simulink model "Composition"  (R2023a)
settings: Solver=FixedStepDiscrete  StartTime=0.0  StopTime=10.0  FixedStep=Ts  RelTol=1e-3
PostLoadFcn:
  | HBridgeCmd_LkupTbl = Simulink.LookupTable;
  | HBridgeCmd_LkupTbl.Table.DataType = 'int16';
  | HBridgeCmd_LkupTbl.Table.Min = [];
  | HBridgeCmd_LkupTbl.Table.Max = [];
  | HBridgeCmd_LkupTbl.Table.Unit = '';
  | HBridgeCmd_LkupTbl.Table.FieldName = 'Table';
  | HBridgeCmd_LkupTbl.Table.Description = '';
  | HBridgeCmd_LkupTbl.Table.Value = int16( ...
  |   [-2048 -1843 -1638 -1434 -1229 -1024 -819 -614 -410 -205 0 205 410 614 ...
  |    819 1024 1229 1434 1638 1843 2048]);
  | HBridgeCmd_LkupTbl.BreakpointsSpecification = 'Explicit values';
  | HBridgeCmd_LkupTbl.SupportTunableSize = false;
  | HBridgeCmd_LkupTbl.Breakpoints.DataType = 'single';
  | HBridgeCmd_LkupTbl.Breakpoints.Min = [];
  | HBridgeCmd_LkupTbl.Breakpoints.Max = [];
  | HBridgeCmd_LkupTbl.Breakpoints.Unit = '';
  | HBridgeCmd_LkupTbl.Breakpoints.FieldName = 'BP1';
  | HBridgeCmd_LkupTbl.Breakpoints.Description = '';
  | HBridgeCmd_LkupTbl.Breakpoints.Value = ...
  |   [-100 -90 -80 -70 -60 -50 -40 -30 -20 -10 0 10 20 30 40 50 60 70 80 90 ...
  |    100];
  | HBridgeCmd_LkupTbl.Breakpoints.TunableSizeName = 'N1';
  | HBridgeCmd_LkupTbl.CoderInfo.StorageClass = 'Auto';
  | HBridgeCmd_LkupTbl.StructTypeInfo.Name = 'MyStruct_Actuator';
  | HBridgeCmd_LkupTbl.StructTypeInfo.DataScope = 'Auto';
  | HBridgeCmd_LkupTbl.StructTypeInfo.HeaderFileName = '';
  | 
  | APP_FilterWeight = Simulink.Parameter;
  | APP_FilterWeight.Value = 1;
  | APP_FilterWeight.CoderInfo.StorageClass = 'Auto';
  | APP_FilterWeight.Description = '';
  | APP_FilterWeight.DataType = 'single';
  | APP_FilterWeight.Min = 0;
  | APP_FilterWeight.Max = 1;
  | APP_FilterWeight.DocUnits = '';
  | 
  | TPS_Primary_FilterWeight = Simulink.Parameter;
  | TPS_Primary_FilterWeight.Value = 1;
  | TPS_Primary_FilterWeight.CoderInfo.StorageClass = 'Auto';
  | TPS_Primary_FilterWeight.Description = '';
  | TPS_Primary_FilterWeight.DataType = 'single';
  | TPS_Primary_FilterWeight.Min = 0;
  | TPS_Primary_FilterWeight.Max = 1;
  | TPS_Primary_FilterWeight.DocUnits = '';
  | 
  | TPS_Secondary_FilterWeight = Simulink.Parameter;
  | TPS_Secondary_FilterWeight.Value = 1;
  | TPS_Secondary_FilterWeight.CoderInfo.StorageClass = 'Auto';
  | TPS_Secondary_FilterWeight.Description = '';
  | TPS_Secondary_FilterWeight.DataType = 'single';
  | TPS_Secondary_FilterWeight.Min = 0;
  | TPS_Secondary_FilterWeight.Max = 1;
  | TPS_Secondary_FilterWeight.DocUnits = '';
  | 
  | AccelPedal_Threshold_High = Simulink.Parameter;
  | AccelPedal_Threshold_High.Value = 975;
  | AccelPedal_Threshold_High.CoderInfo.StorageClass = 'Auto';
  | AccelPedal_Threshold_High.Description = '';
  | AccelPedal_Threshold_High.DataType = 'uint16';
  | AccelPedal_Threshold_High.Min = 0;
  | AccelPedal_Threshold_High.Max = 1023;
  | AccelPedal_Threshold_High.DocUnits = '';
  | 
  | AccelPedal_Threshold_Low = Simulink.Parameter;
  | AccelPedal_Threshold_Low.Value = 50;
  | AccelPedal_Threshold_Low.CoderInfo.StorageClass = 'Auto';
  | AccelPedal_Threshold_Low.Description = '';
  | AccelPedal_Threshold_Low.DataType = 'uint16';
  | AccelPedal_Threshold_Low.Min = 0;
  | AccelPedal_Threshold_Low.Max = 1023;
  | AccelPedal_Threshold_Low.DocUnits = '';
  | 
  | TPS_Primary_Threshold_High = Simulink.Parameter;
  | TPS_Primary_Threshold_High.Value = 975;
  | TPS_Primary_Threshold_High.CoderInfo.StorageClass = 'Auto';
  | TPS_Primary_Threshold_High.Description = '';
  | TPS_Primary_Threshold_High.DataType = 'uint16';
  | TPS_Primary_Threshold_High.Min = 0;
  | TPS_Primary_Threshold_High.Max = 1023;
  | TPS_Primary_Threshold_High.DocUnits = '';
  | 
  | TPS_Primary_Threshold_Low = Simulink.Parameter;
  | TPS_Primary_Threshold_Low.Value = 50;
  | TPS_Primary_Threshold_Low.CoderInfo.StorageClass = 'Auto';
  | TPS_Primary_Threshold_Low.Description = '';
  | TPS_Primary_Threshold_Low.DataType = 'uint16';
  | TPS_Primary_Threshold_Low.Min = 0;
  | TPS_Primary_Threshold_Low.Max = 1023;
  | TPS_Primary_Threshold_Low.DocUnits = '';
  | 
  | TPS_Secondary_Threshold_High = Simulink.Parameter;
  | TPS_Secondary_Threshold_High.Value = 975;
  | TPS_Secondary_Threshold_High.CoderInfo.StorageClass = 'Auto';
  | TPS_Secondary_Threshold_High.Description = '';
  | TPS_Secondary_Threshold_High.DataType = 'uint16';
  | TPS_Secondary_Threshold_High.Min = 0;
  | TPS_Secondary_Threshold_High.Max = 1023;
  | TPS_Secondary_Threshold_High.DocUnits = '';
  | 
  | TPS_Secondary_Threshold_Low = Simulink.Parameter;
  | TPS_Secondary_Threshold_Low.Value = 50;
  | TPS_Secondary_Threshold_Low.CoderInfo.StorageClass = 'Auto';
  | TPS_Secondary_Threshold_Low.Description = '';
  | TPS_Secondary_Threshold_Low.DataType = 'uint16';
  | TPS_Secondary_Threshold_Low.Min = 0;
  | TPS_Secondary_Threshold_Low.Max = 1023;
  | TPS_Secondary_Threshold_Low.DocUnits = '';
  | 
  | 
  | SetpointPercent_LkupTbl = Simulink.LookupTable;
  | SetpointPercent_LkupTbl.Table.DataType = 'single';
  | SetpointPercent_LkupTbl.Table.Min = [];
  | SetpointPercent_LkupTbl.Table.Max = [];
  | SetpointPercent_LkupTbl.Table.Unit = '';
  | SetpointPercent_LkupTbl.Table.FieldName = 'Table';
  | SetpointPercent_LkupTbl.Table.Description = '';
  | SetpointPercent_LkupTbl.Table.Value = ...
  |   [0 10 20 30 40 50 60 70 80 90 100];
  | SetpointPercent_LkupTbl.BreakpointsSpecification = 'Explicit values';
  | SetpointPercent_LkupTbl.SupportTunableSize = false;
  | SetpointPercent_LkupTbl.Breakpoints.DataType = 'single';
  | SetpointPercent_LkupTbl.Breakpoints.Min = [];
  | SetpointPercent_LkupTbl.Breakpoints.Max = [];
  | SetpointPercent_LkupTbl.Breakpoints.Unit = '';
  | SetpointPercent_LkupTbl.Breakpoints.FieldName = 'BP1';
  | SetpointPercent_LkupTbl.Breakpoints.Description = '';
  | SetpointPercent_LkupTbl.Breakpoints.Value = ...
  |   [0 100 200 300 400 500 600 700 800 900 1000];
  | SetpointPercent_LkupTbl.Breakpoints.TunableSizeName = 'N1';
  | SetpointPercent_LkupTbl.CoderInfo.StorageClass = 'Auto';
  | SetpointPercent_LkupTbl.StructTypeInfo.Name = 'MyStruct';
  | SetpointPercent_LkupTbl.StructTypeInfo.DataScope = 'Auto';
  | SetpointPercent_LkupTbl.StructTypeInfo.HeaderFileName = '';
  | 
  | TPSPrimaryPercent_LkupTbl = Simulink.LookupTable;
  | TPSPrimaryPercent_LkupTbl.Table.DataType = 'single';
  | TPSPrimaryPercent_LkupTbl.Table.Min = [];
  | TPSPrimaryPercent_LkupTbl.Table.Max = [];
  | TPSPrimaryPercent_LkupTbl.Table.Unit = '';
  | TPSPrimaryPercent_LkupTbl.Table.FieldName = 'Table';
  | TPSPrimaryPercent_LkupTbl.Table.Description = '';
  | TPSPrimaryPercent_LkupTbl.Table.Value = ...
  |   [0 10 20 30 40 50 60 70 80 90 100];
  | TPSPrimaryPercent_LkupTbl.BreakpointsSpecification = 'Explicit values';
  | TPSPrimaryPercent_LkupTbl.SupportTunableSize = false;
  | TPSPrimaryPercent_LkupTbl.Breakpoints.DataType = 'single';
  | TPSPrimaryPercent_LkupTbl.Breakpoints.Min = [];
  | TPSPrimaryPercent_LkupTbl.Breakpoints.Max = [];
  | TPSPrimaryPercent_LkupTbl.Breakpoints.Unit = '';
  | TPSPrimaryPercent_LkupTbl.Breakpoints.FieldName = 'BP1';
  | TPSPrimaryPercent_LkupTbl.Breakpoints.Description = '';
  | TPSPrimaryPercent_LkupTbl.Breakpoints.Value = ...
  |   [0 100 200 300 400 500 600 700 800 900 1000];
  | TPSPrimaryPercent_LkupTbl.Breakpoints.TunableSizeName = 'N1';
  | TPSPrimaryPercent_LkupTbl.CoderInfo.StorageClass = 'Auto';
  | TPSPrimaryPercent_LkupTbl.StructTypeInfo.Name = 'MyStruct';
  | TPSPrimaryPercent_LkupTbl.StructTypeInfo.DataScope = 'Auto';
  | TPSPrimaryPercent_LkupTbl.StructTypeInfo.HeaderFileName = '';
  | 
  | TPSSecondaryPercent_LkupTbl = Simulink.LookupTable;
  | TPSSecondaryPercent_LkupTbl.Table.DataType = 'single';
  | TPSSecondaryPercent_LkupTbl.Table.Min = [];
  | TPSSecondaryPercent_LkupTbl.Table.Max = [];
  | TPSSecondaryPercent_LkupTbl.Table.Unit = '';
  | TPSSecondaryPercent_LkupTbl.Table.FieldName = 'Table';
  | TPSSecondaryPercent_LkupTbl.Table.Description = '';
  | TPSSecondaryPercent_LkupTbl.Table.Value = ...
  |   [100 90 80 70 60 50 40 30 20 10 0];
  | TPSSecondaryPercent_LkupTbl.BreakpointsSpecification = ...
  |   'Explicit values';
  | TPSSecondaryPercent_LkupTbl.SupportTunableSize = false;
  | TPSSecondaryPercent_LkupTbl.Breakpoints.DataType = 'single';
  | TPSSecondaryPercent_LkupTbl.Breakpoints.Min = [];
  | TPSSecondaryPercent_LkupTbl.Breakpoints.Max = [];
  | TPSSecondaryPercent_LkupTbl.Breakpoints.Unit = '';
  | TPSSecondaryPercent_LkupTbl.Breakpoints.FieldName = 'BP1';
  | TPSSecondaryPercent_LkupTbl.Breakpoints.Description = '';
  | TPSSecondaryPercent_LkupTbl.Breakpoints.Value = ...
  |   [0 100 200 300 400 500 600 700 800 900 1000];
  | TPSSecondaryPercent_LkupTbl.Breakpoints.TunableSizeName = 'N1';
  | TPSSecondaryPercent_LkupTbl.CoderInfo.StorageClass = 'Auto';
  | TPSSecondaryPercent_LkupTbl.StructTypeInfo.Name = 'MyStruct';
  | TPSSecondaryPercent_LkupTbl.StructTypeInfo.DataScope = 'Auto';
  | TPSSecondaryPercent_LkupTbl.StructTypeInfo.HeaderFileName = '';
  | 
  | Ts = 0.005;
undefined symbols (not defined in the file): D1, P
CloseFcn:
  | clear Ts TPSSecondaryPercent_LkupTbl TPSPrimaryPercent_LkupTbl SetpointPercent_LkupTbl ...
  |     TPS_Secondary_Threshold_High TPS_Secondary_Threshold_Low ...
  |     TPS_Primary_Threshold_High TPS_Primary_Threshold_Low ...
  |     TPS_Primary_FilterWeight TPS_Secondary_FilterWeight ...
  |     AccelPedal_Threshold_High AccelPedal_Threshold_Low ...
  |     APP_FilterWeight HBridgeCmd_LkupTbl
settings Model: Creator=The MathWorks, Inc.  LastModifiedBy=omert
settings OptimizationCC: DefaultParameterBehavior=Inlined  EnhancedBackFolding=on  PassReuseOutputArgsAs=Individual arguments  ZeroExternalMemoryAtStartup=off  ZeroInternalMemoryAtStartup=off  OptimizeBlockOrder=speed  DifferentSizesBufferReuse=on  OptimizationCustomize=off  EfficientTunableParamExpr=on
settings DebuggingCC: ParameterTunabilityLossMsg=error  UnconnectedInputMsg=warning  UnconnectedOutputMsg=warning  UnconnectedLineMsg=warning
settings ModelReferenceCC: EnableRefExpFcnMdlSchedulingChecks=on
settings SFSimCC: MATLABDynamicMemAlloc=off
settings RTWCC: Description=Embedded Coder  SystemTargetFile=ert.tlc  TemplateMakefile=ert_default_tmf  DLArmComputeVersion=19.05
settings CodeAppCC: ForceParamTrailComments=on  IgnoreCustomStorageClasses=off  MaxIdLength=255  OperatorAnnotations=on  SimulinkDataObjDesc=on  SFDataObjDesc=on  InsertBlockDesc=on
settings ERTTargetCC: TargetLangStandard=C99 (ISO)  GenerateSampleERTMain=on  InlinedParameterPlacement=NonHierarchical  ERTCustomFileTemplate=example_file_process.tlc

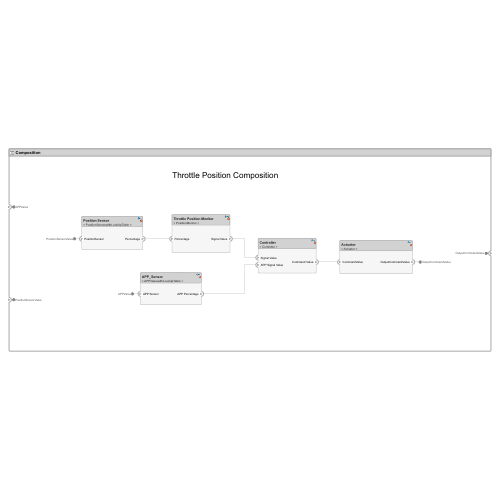
[thumbnail: Simulink's stored preview of the top-level diagram]
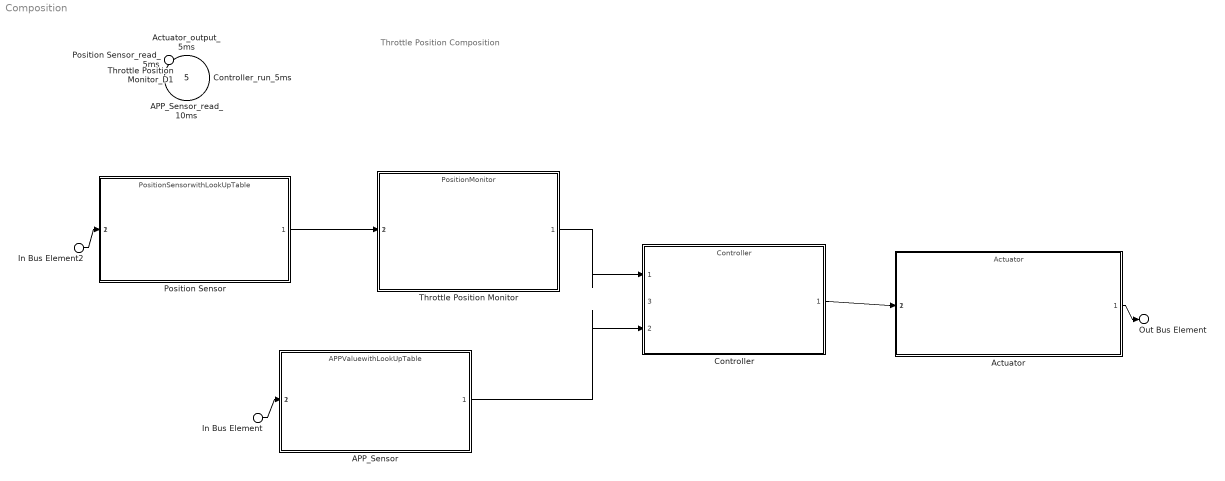
== system Composition ==
  note: Throttle Position Composition
  In Bus Element : Inport  PortName=APPValue
  In Bus Element2 : Inport  Port=2  PortName=PositionSensorValue
  APP_Sensor_read_10ms : Inport  Port=3  OutputFunctionCall=on
  Actuator_output_5ms : Inport  Port=4  OutputFunctionCall=on
  Controller_run_5ms : Inport  Port=5  OutputFunctionCall=on
  Position Sensor_read_5ms : Inport  Port=6  OutputFunctionCall=on
  Throttle Position Monitor_D1 : Inport  Port=7  OutputFunctionCall=on
  APP_Sensor : ModelReference  ModelNameDialog=APPValuewithLookUpTable  SimulationMode=Normal  ScheduleRates=on  ModelReferenceVersion=5.2
      settings: PortSchema="{\"entries\":[{\"content\":{\"headerSize\":38,\"margin\":15,\"minimumSpacing\":25,\"sides\":[{\"content\":{\"connectorIds\":[\"In1\"]},\"type\":\"ConnectorPlacement.EquallySpacedRectSide\",\"uuid\":\"c29aa152-21e6-4ee4-993c-b72c52d53eaf\"},{\"content\":{\"connectorIds\":[\"Out1\"],\"side\":\"RIGHT\"},\"type\":\"ConnectorPlacement.EquallySpacedRectSide\",\"uuid\":\"9c4e8262-d4f5-4a71-85d6-4174f9813a5f\"},{\"content\":{\"connectorIds\":[],\"side\":\"TOP\"},\"type\":\"ConnectorPlacement.EquallySpacedRectSide\",\"uuid\":\"c9ef3685-fbcc-4180-9c44-6a6e7c5f1244\"},{\"content\":{\"connectorIds\":[\"In2\"],\"side\":\"HIDDEN\"},\"type\":\"ConnectorPlacement.EquallySpacedRectSide\",\"uuid\":\"f1270cb8-53b9-476f-b22e-76ae4b133e3f\"}]},\"type\":\"ConnectorPlacement.EquallySpacedConnector\",\"uuid\":\"93ccf44c-7afb-4857-9748-e933214d86ea\"}],\"packageUris\":[\"http://schema.mathworks.com/mf0/Connector/R2020b\"],\"version\":\"1.0\"}"
  Actuator : ModelReference  ModelNameDialog=Actuator  SimulationMode=Normal  ScheduleRates=on  ModelReferenceVersion=5.2
      settings: PortSchema="{\"entries\":[{\"content\":{\"headerSize\":38,\"margin\":15,\"minimumSpacing\":25,\"sides\":[{\"content\":{\"connectorIds\":[\"In1\"]},\"type\":\"ConnectorPlacement.EquallySpacedRectSide\",\"uuid\":\"c29aa152-21e6-4ee4-993c-b72c52d53eaf\"},{\"content\":{\"connectorIds\":[\"Out1\"],\"side\":\"RIGHT\"},\"type\":\"ConnectorPlacement.EquallySpacedRectSide\",\"uuid\":\"9c4e8262-d4f5-4a71-85d6-4174f9813a5f\"},{\"content\":{\"connectorIds\":[],\"side\":\"TOP\"},\"type\":\"ConnectorPlacement.EquallySpacedRectSide\",\"uuid\":\"c9ef3685-fbcc-4180-9c44-6a6e7c5f1244\"},{\"content\":{\"connectorIds\":[\"In2\"],\"side\":\"HIDDEN\"},\"type\":\"ConnectorPlacement.EquallySpacedRectSide\",\"uuid\":\"00201e36-4798-4d6f-9c06-922f886f8b8e\"}]},\"type\":\"ConnectorPlacement.EquallySpacedConnector\",\"uuid\":\"93ccf44c-7afb-4857-9748-e933214d86ea\"}],\"packageUris\":[\"http://schema.mathworks.com/mf0/Connector/R2020b\"],\"version\":\"1.0\"}"
  Controller : ModelReference  ModelNameDialog=Controller  SimulationMode=Normal  ScheduleRates=on  ModelReferenceVersion=5.4
      settings: PortSchema="{\"entries\":[{\"content\":{\"headerSize\":38,\"margin\":15,\"minimumSpacing\":25,\"sides\":[{\"content\":{\"connectorIds\":[\"In1\",\"In2\"]},\"type\":\"ConnectorPlacement.EquallySpacedRectSide\",\"uuid\":\"c29aa152-21e6-4ee4-993c-b72c52d53eaf\"},{\"content\":{\"connectorIds\":[\"Out1\"],\"side\":\"RIGHT\"},\"type\":\"ConnectorPlacement.EquallySpacedRectSide\",\"uuid\":\"9c4e8262-d4f5-4a71-85d6-4174f9813a5f\"},{\"content\":{\"connectorIds\":[],\"side\":\"TOP\"},\"type\":\"ConnectorPlacement.EquallySpacedRectSide\",\"uuid\":\"c9ef3685-fbcc-4180-9c44-6a6e7c5f1244\"},{\"content\":{\"connectorIds\":[\"In3\"],\"side\":\"HIDDEN\"},\"type\":\"ConnectorPlacement.EquallySpacedRectSide\",\"uuid\":\"cd41997d-1e34-4368-8511-2b1fe694f98a\"}]},\"type\":\"ConnectorPlacement.EquallySpacedConnector\",\"uuid\":\"93ccf44c-7afb-4857-9748-e933214d86ea\"}],\"packageUris\":[\"http://schema.mathworks.com/mf0/Connector/R2020b\"],\"version\":\"1.0\"}"
  Position Sensor : ModelReference  ModelNameDialog=PositionSensorwithLookUpTable  UsingDefaultArgumentValue=0  SimulationMode=Normal  ScheduleRates=on  ModelReferenceVersion=5.3
      settings: PortSchema="{\"entries\":[{\"content\":{\"headerSize\":38,\"margin\":15,\"minimumSpacing\":25,\"sides\":[{\"content\":{\"connectorIds\":[\"In1\"]},\"type\":\"ConnectorPlacement.EquallySpacedRectSide\",\"uuid\":\"c29aa152-21e6-4ee4-993c-b72c52d53eaf\"},{\"content\":{\"connectorIds\":[\"Out1\"],\"side\":\"RIGHT\"},\"type\":\"ConnectorPlacement.EquallySpacedRectSide\",\"uuid\":\"9c4e8262-d4f5-4a71-85d6-4174f9813a5f\"},{\"content\":{\"connectorIds\":[],\"side\":\"TOP\"},\"type\":\"ConnectorPlacement.EquallySpacedRectSide\",\"uuid\":\"c9ef3685-fbcc-4180-9c44-6a6e7c5f1244\"},{\"content\":{\"connectorIds\":[\"In2\"],\"side\":\"HIDDEN\"},\"type\":\"ConnectorPlacement.EquallySpacedRectSide\",\"uuid\":\"9e42063d-e5ff-4629-a071-cb979e3a0f50\"}]},\"type\":\"ConnectorPlacement.EquallySpacedConnector\",\"uuid\":\"93ccf44c-7afb-4857-9748-e933214d86ea\"}],\"packageUris\":[\"http://schema.mathworks.com/mf0/Connector/R2020b\"],\"version\":\"1.0\"}"
  Throttle Position Monitor : ModelReference  ModelNameDialog=PositionMonitor  SimulationMode=Normal  ScheduleRates=on  CachedPortDiscreteRates=[0.005]  ModelEventPortInfo=P:D1[0.005][0][0]  ModelReferenceVersion=5.2
      settings: PortSchema="{\"entries\":[{\"content\":{\"headerSize\":38,\"margin\":15,\"minimumSpacing\":25,\"sides\":[{\"content\":{\"connectorIds\":[\"In1\"]},\"type\":\"ConnectorPlacement.EquallySpacedRectSide\",\"uuid\":\"c29aa152-21e6-4ee4-993c-b72c52d53eaf\"},{\"content\":{\"connectorIds\":[\"Out1\"],\"side\":\"RIGHT\"},\"type\":\"ConnectorPlacement.EquallySpacedRectSide\",\"uuid\":\"9c4e8262-d4f5-4a71-85d6-4174f9813a5f\"},{\"content\":{\"side\":\"TOP\"},\"type\":\"ConnectorPlacement.EquallySpacedRectSide\",\"uuid\":\"c9ef3685-fbcc-4180-9c44-6a6e7c5f1244\"},{\"content\":{\"connectorIds\":[\"In2\"],\"side\":\"HIDDEN\"},\"type\":\"ConnectorPlacement.EquallySpacedRectSide\",\"uuid\":\"a46fe878-a4a6-4148-b4e0-a6c758e9fec2\"}]},\"type\":\"ConnectorPlacement.EquallySpacedConnector\",\"uuid\":\"93ccf44c-7afb-4857-9748-e933214d86ea\"}],\"packageUris\":[\"http://schema.mathworks.com/mf0/Connector/R2020b\"],\"version\":\"1.0\"}"
  Out Bus Element : Outport  PortName=OutputCommandValue
  wires:
  In Bus Element/1 -> APP_Sensor/1
  In Bus Element2/1 -> Position Sensor/1
  APP_Sensor/1 -> Controller/2
  Actuator/1 -> Out Bus Element/1
  Controller/1 -> Actuator/1
  Position Sensor/1 -> Throttle Position Monitor/1
  Throttle Position Monitor/1 -> Controller/1
